simulink library "lib_rigidbody_dynamics_mapletb_mod"  (Simulink 8.5)
settings: Solver=ode45  StartTime=0.0  StopTime=10.0  RelTol=1e-3
undefined symbols (not defined in the file or in its folder): DynPar1, NJ, phi_base_t0, rpy2r, rpyD2omega
undefined symbols (not defined in the file): g_W, KinPar_mdh, phiD_base_t0, r_t0, rD_t0
libraries: transformations_lib x4, rigid_body_kinematics x2
settings Model: Creator=schappler  LastModifiedBy=schappler

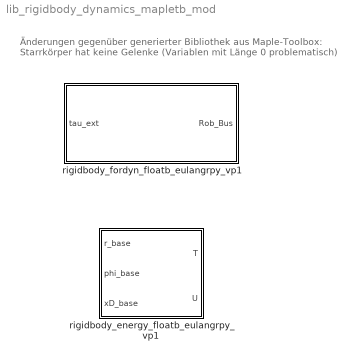
== system lib_rigidbody_dynamics_mapletb_mod ==
  note: Änderungen gegenüber generierter Bibliothek aus Maple-Toolbox:
      | Starrkörper hat keine Gelenke (Variablen mit Länge 0 problematisch)
  rigidbody_energy_floatb_eulangrpy_vp1 : Subsystem  mask{KinPar_mdh=KinPar_mdh, DynPar1=DynPar1, g_world=g_W}
      mask prompts: KinPar_mdh "Kinematik-Parameter"; DynPar1 "Dynamik-Parameter (Parametersatz 1)"; g_world "Gravitationsvektor im Welt-KS (g_world)"
  rigidbody_fordyn_floatb_eulangrpy_vp1 : Subsystem  mask{r_base_t0=r_t0, rD_base_t0=rD_t0, phi_base_t0=phi_base_t0, phiD_base_t0=phiD_base_t0, g_world=g_W, KinPar_mdh=KinPar_mdh, DynPar1=DynPar1}
      mask prompts: r_base_t0 "r_base_t0 (Basisposition im Welt-KS)"; KinPar_mdh "Kinematik-Parameter"; DynPar1 "Dynamik-Parameter (Parametersatz 1)"
      mask Display:
      | port_label('input', 1, '_{(W)} F^{ext}', 'texmode', 'on')
      | port_label('output', 1, 'Rob_Bus')

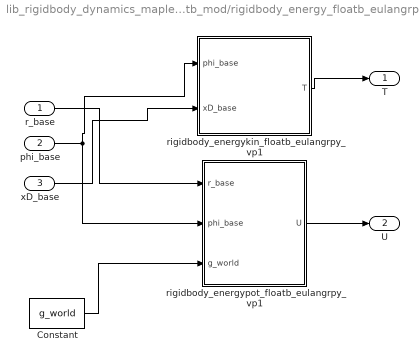
== system lib_rigidbody_dynamics_mapletb_mod/rigidbody_energy_floatb_eulangrpy_vp1 ==
  r_base : Inport
  phi_base : Inport  Port=2
  xD_base : Inport  Port=3
  Constant : Constant  Value=g_world
  rigidbody_energykin_floatb_eulangrpy_vp1 : Subsystem  mask{KinPar_mdh=KinPar_mdh, DynPar1=DynPar1}
      mask prompts: KinPar_mdh "Kinematik-Parameter"; DynPar1 "Dynamik-Parameter (Parametersatz 1)"
      mask init:
      | a_mdh = KinPar_mdh.a;
      | d_mdh = KinPar_mdh.d;
      | b_mdh = KinPar_mdh.b;
      | beta_mdh = KinPar_mdh.beta;
      | alpha_mdh = KinPar_mdh.alpha;
      | q_offset_mdh = KinPar_mdh.q_offset;
      | 
      | m = DynPar1.m;
      | r_S = DynPar1.r_S;
      | I_S = DynPar1.I_S;
  rigidbody_energypot_floatb_eulangrpy_vp1 : Subsystem  mask{KinPar_mdh=KinPar_mdh, DynPar1=DynPar1}
      mask prompts: KinPar_mdh "Kinematik-Parameter"; DynPar1 "Dynamik-Parameter (Parametersatz 1)"
      mask init: same as lib_rigidbody_dynamics_mapletb_mod/rigidbody_energy_floatb_eulangrpy_vp1/rigidbody_energykin_floatb_eulangrpy_vp1
  T : Outport
  U : Outport  Port=2
  wires:
  Constant/1 -> rigidbody_energypot_floatb_eulangrpy_vp1/3(g_world)
  rigidbody_energypot_floatb_eulangrpy_vp1/1(U) -> U/1
  rigidbody_energykin_floatb_eulangrpy_vp1/1(T) -> T/1
  phi_base/1 -> rigidbody_energykin_floatb_eulangrpy_vp1/1(phi_base), rigidbody_energypot_floatb_eulangrpy_vp1/2(phi_base)
  r_base/1 -> rigidbody_energypot_floatb_eulangrpy_vp1/1(r_base)
  xD_base/1 -> rigidbody_energykin_floatb_eulangrpy_vp1/2(xD_base)

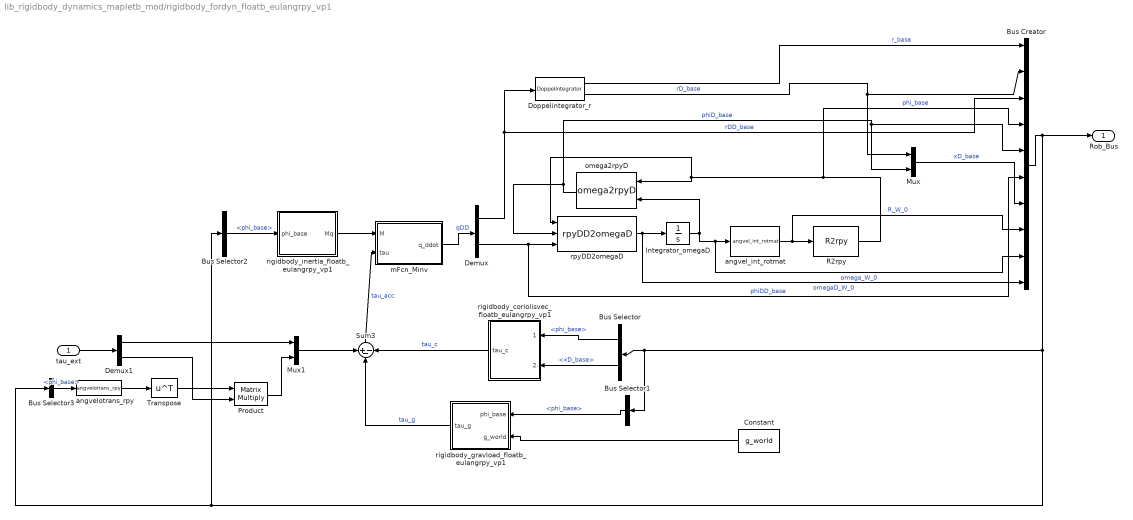
== system lib_rigidbody_dynamics_mapletb_mod/rigidbody_fordyn_floatb_eulangrpy_vp1 ==
  "tau_ext " : Inport  PortDimensions=6+NJ
  Bus Creator : BusCreator  Inputs=10
  Bus Selector : BusSelector  OutputSignals=phi_base,xD_base
  Bus Selector1 : BusSelector  OutputSignals=phi_base
  Bus Selector2 : BusSelector  OutputSignals=phi_base
  Bus Selector3 : BusSelector  OutputSignals=phi_base
  Constant : Constant  Value=g_world
  Demux : Demux  Outputs=[3 3]
  Demux1 : Demux  Outputs=[3 3]
  Doppelintegrator_r : rigid_body_kinematics/Doppelintegrator  r0=r_base_t0  rD0=rD_base_t0  Name_v='x'
  Integrator_omegaD : Integrator  InitialCondition=rpyD2omega(phi_base_t0', phiD_base_t0')'
  Mux : Mux  Inputs=2
  Mux1 : Mux  Inputs=2
  Product : Product  Multiplication=Matrix(*)
  R2rpy : transformations_lib/R2rpy
  Sum3 : Sum  Inputs=+--
  Transpose : Math  Operator=transpose  SaturateOnIntegerOverflow=on
  angvel_int_rotmat : rigid_body_kinematics/angvel_int_rotmat  R_0E_t0=rpy2r(phi_base_t0(1), phi_base_t0(2), phi_base_t0(3) )
  angvelotrans_rpy : transformations_lib/angvelotrans_rpy
  mFcn_Minv : MATLAB Function  TreatAsAtomicUnit=on
  omega2rpyD : transformations_lib/omega2rpyD
  rigidbody_coriolisvec_floatb_eulangrpy_vp1 : Subsystem  mask{KinPar_mdh=KinPar_mdh, DynPar1=DynPar1}
      mask prompts: KinPar_mdh "Kinematik-Parameter"; DynPar1 "Dynamik-Parameter (Parametersatz 1)"
      mask init: same as lib_rigidbody_dynamics_mapletb_mod/rigidbody_energy_floatb_eulangrpy_vp1/rigidbody_energykin_floatb_eulangrpy_vp1
  rigidbody_gravload_floatb_eulangrpy_vp1 : Subsystem  mask{KinPar_mdh=KinPar_mdh, DynPar1=DynPar1}
      mask prompts: KinPar_mdh "Kinematik-Parameter"; DynPar1 "Dynamik-Parameter (Parametersatz 1)"
      mask init: same as lib_rigidbody_dynamics_mapletb_mod/rigidbody_energy_floatb_eulangrpy_vp1/rigidbody_energykin_floatb_eulangrpy_vp1
  rigidbody_inertia_floatb_eulangrpy_vp1 : Subsystem  mask{KinPar_mdh=KinPar_mdh, DynPar1=DynPar1}
      mask prompts: KinPar_mdh "Kinematik-Parameter"; DynPar1 "Dynamik-Parameter (Parametersatz 1)"
      mask init: same as lib_rigidbody_dynamics_mapletb_mod/rigidbody_energy_floatb_eulangrpy_vp1/rigidbody_energykin_floatb_eulangrpy_vp1
  rpyDD2omegaD : transformations_lib/rpyDD2omegaD
  Rob_Bus : Outport
  wires:
  Bus Selector2/1 -> rigidbody_inertia_floatb_eulangrpy_vp1/1(phi_base)  "<phi_base>"
  Bus Selector1/1 -> rigidbody_gravload_floatb_eulangrpy_vp1/1(phi_base)  "<phi_base>"
  Bus Selector/1 -> rigidbody_coriolisvec_floatb_eulangrpy_vp1/1(phi_base)  "<phi_base>"
  Bus Selector/2 -> rigidbody_coriolisvec_floatb_eulangrpy_vp1/2(xD_base)  "<xD_base>"
  Bus Creator/1 -> Rob_Bus/1, Bus Selector/1, Bus Selector1/1, Bus Selector3/1, Bus Selector2/1
  Mux/1 -> Bus Creator/7  "xD_base"
  Doppelintegrator_r/2 -> Bus Creator/2, Mux/1  "rD_base"
  Doppelintegrator_r/1 -> Bus Creator/1  "r_base"
  omega2rpyD/1 -> Bus Creator/5, Mux/2, rpyDD2omegaD/2  "phiD_base"
  R2rpy/1 -> omega2rpyD/1, rpyDD2omegaD/1, Bus Creator/4  "phi_base"
  angvel_int_rotmat/1 -> Bus Creator/8, R2rpy/1  "R_W_0"
  Demux/2 -> Bus Creator/6, rpyDD2omegaD/3  "phiDD_base"
  Integrator_omegaD/1 -> Bus Creator/9, angvel_int_rotmat/1, omega2rpyD/2  "omega_W_0"
  rpyDD2omegaD/1 -> Integrator_omegaD/1, Bus Creator/10  "omegaD_W_0"
  Demux/1 -> Doppelintegrator_r/1, Bus Creator/3  "rDD_base"
  rigidbody_gravload_floatb_eulangrpy_vp1/1(tau_g) -> Sum3/2  "tau_g"
  mFcn_Minv/1(q_ddot) -> Demux/1  "qDD"
  rigidbody_coriolisvec_floatb_eulangrpy_vp1/1(tau_c) -> Sum3/3  "tau_c"
  "tau_ext "/1 -> Demux1/1
  Sum3/1 -> mFcn_Minv/2(tau)  "tau_acc"
  rigidbody_inertia_floatb_eulangrpy_vp1/1(Mq) -> mFcn_Minv/1(M)
  Constant/1 -> rigidbody_gravload_floatb_eulangrpy_vp1/2(g_world)
  Demux1/2 -> Product/2
  Demux1/1 -> Mux1/1
  Bus Selector3/1 -> angvelotrans_rpy/1  "<phi_base>"
  angvelotrans_rpy/1 -> Transpose/1
  Product/1 -> Mux1/2
  Mux1/1 -> Sum3/1
  Transpose/1 -> Product/1

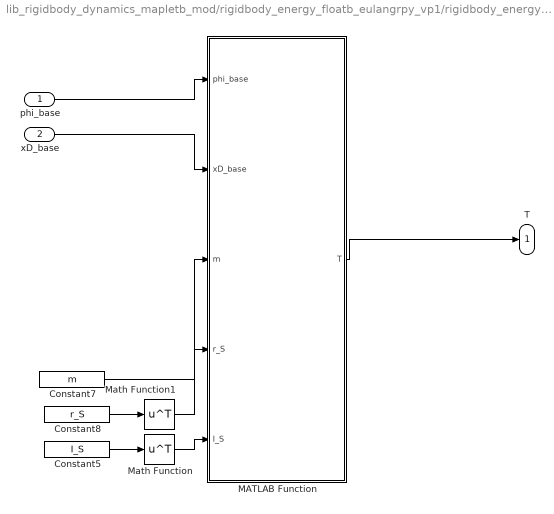
== system lib_rigidbody_dynamics_mapletb_mod/rigidbody_energy_floatb_eulangrpy_vp1/rigidbody_energykin_floatb_eulangrpy_vp1 ==
  phi_base : Inport
  xD_base : Inport  Port=2
  Constant5 : Constant  Value=I_S
  Constant7 : Constant  Value=m
  Constant8 : Constant  Value=r_S
  MATLAB Function : MATLAB Function  TreatAsAtomicUnit=on
  Math Function : Math  Operator=transpose  SaturateOnIntegerOverflow=on
  Math Function1 : Math  Operator=transpose  SaturateOnIntegerOverflow=on
  T : Outport
  wires:
  xD_base/1 -> MATLAB Function/2(xD_base)
  phi_base/1 -> MATLAB Function/1(phi_base)
  Constant5/1 -> Math Function/1
  Constant8/1 -> Math Function1/1
  Constant7/1 -> MATLAB Function/3(m)
  MATLAB Function/1(T) -> T/1
  Math Function/1 -> MATLAB Function/5(I_S)
  Math Function1/1 -> MATLAB Function/4(r_S)

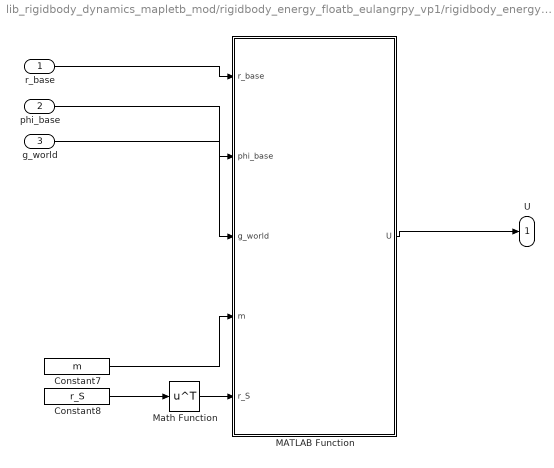
== system lib_rigidbody_dynamics_mapletb_mod/rigidbody_energy_floatb_eulangrpy_vp1/rigidbody_energypot_floatb_eulangrpy_vp1 ==
  r_base : Inport
  phi_base : Inport  Port=2
  g_world : Inport  Port=3
  Constant7 : Constant  Value=m
  Constant8 : Constant  Value=r_S
  MATLAB Function : MATLAB Function  TreatAsAtomicUnit=on
  Math Function : Math  Operator=transpose  SaturateOnIntegerOverflow=on
  U : Outport
  wires:
  phi_base/1 -> MATLAB Function/2(phi_base)
  r_base/1 -> MATLAB Function/1(r_base)
  Constant8/1 -> Math Function/1
  Constant7/1 -> MATLAB Function/4(m)
  g_world/1 -> MATLAB Function/3(g_world)
  MATLAB Function/1(U) -> U/1
  Math Function/1 -> MATLAB Function/5(r_S)

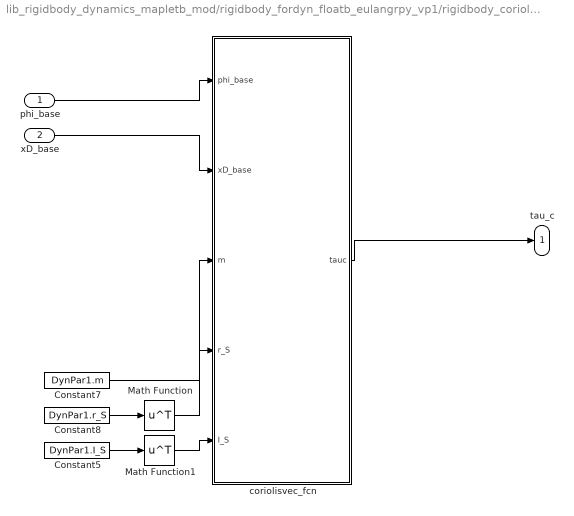
== system lib_rigidbody_dynamics_mapletb_mod/rigidbody_fordyn_floatb_eulangrpy_vp1/rigidbody_coriolisvec_floatb_eulangrpy_vp1 ==
  phi_base : Inport
  xD_base : Inport  Port=2
  Constant5 : Constant  Value=DynPar1.I_S
  Constant7 : Constant  Value=DynPar1.m
  Constant8 : Constant  Value=DynPar1.r_S
  Math Function : Math  Operator=transpose  SaturateOnIntegerOverflow=on
  Math Function1 : Math  Operator=transpose  SaturateOnIntegerOverflow=on
  coriolisvec_fcn : MATLAB Function  TreatAsAtomicUnit=on
  tau_c : Outport
  wires:
  xD_base/1 -> coriolisvec_fcn/2(xD_base)
  phi_base/1 -> coriolisvec_fcn/1(phi_base)
  Constant5/1 -> Math Function1/1
  Constant8/1 -> Math Function/1
  Constant7/1 -> coriolisvec_fcn/3(m)
  coriolisvec_fcn/1(tauc) -> tau_c/1
  Math Function/1 -> coriolisvec_fcn/4(r_S)
  Math Function1/1 -> coriolisvec_fcn/5(I_S)

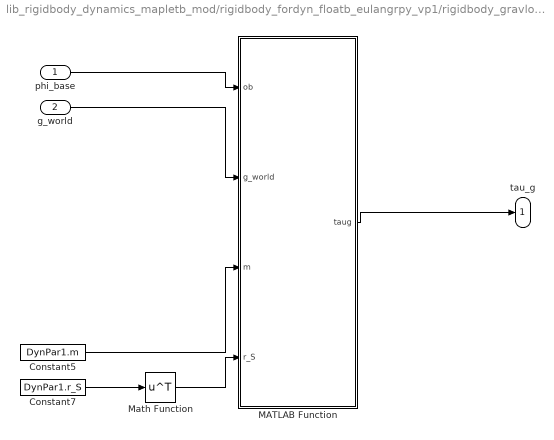
== system lib_rigidbody_dynamics_mapletb_mod/rigidbody_fordyn_floatb_eulangrpy_vp1/rigidbody_gravload_floatb_eulangrpy_vp1 ==
  phi_base : Inport
  g_world : Inport  Port=2
  Constant5 : Constant  Value=DynPar1.m
  Constant7 : Constant  Value=DynPar1.r_S
  MATLAB Function : MATLAB Function  TreatAsAtomicUnit=on
  Math Function : Math  Operator=transpose  SaturateOnIntegerOverflow=on
  tau_g : Outport
  wires:
  phi_base/1 -> MATLAB Function/1(ob)
  Constant7/1 -> Math Function/1
  Constant5/1 -> MATLAB Function/3(m)
  g_world/1 -> MATLAB Function/2(g_world)
  MATLAB Function/1(taug) -> tau_g/1
  Math Function/1 -> MATLAB Function/4(r_S)

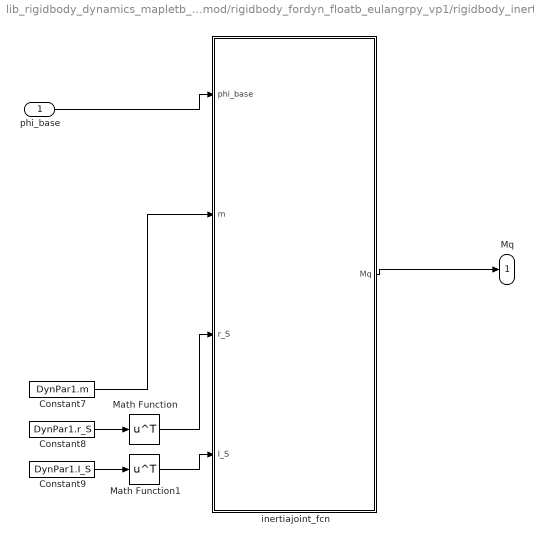
== system lib_rigidbody_dynamics_mapletb_mod/rigidbody_fordyn_floatb_eulangrpy_vp1/rigidbody_inertia_floatb_eulangrpy_vp1 ==
  phi_base : Inport
  Constant7 : Constant  Value=DynPar1.m
  Constant8 : Constant  Value=DynPar1.r_S
  Constant9 : Constant  Value=DynPar1.I_S
  Math Function : Math  Operator=transpose  SaturateOnIntegerOverflow=on
  Math Function1 : Math  Operator=transpose  SaturateOnIntegerOverflow=on
  inertiajoint_fcn : MATLAB Function  TreatAsAtomicUnit=on
  Mq : Outport
  wires:
  phi_base/1 -> inertiajoint_fcn/1(phi_base)
  Constant9/1 -> Math Function1/1
  Constant8/1 -> Math Function/1
  inertiajoint_fcn/1(Mq) -> Mq/1
  Constant7/1 -> inertiajoint_fcn/2(m)
  Math Function/1 -> inertiajoint_fcn/3(r_S)
  Math Function1/1 -> inertiajoint_fcn/4(I_S)

== matlab function rigidbody_fordyn_floatb_eulangrpy_vp1/rigidbody_gravload_floatb_eulangrpy_vp1/MATLAB Function ==
  data: taug output double; ob input double; g_world input double; m input double; r_S input double
function taug = gravload(ob, g_world, ...
  m, r_S)
%#codegen
q = zeros(0,1);
alpha_mdh = zeros(0,1);
a_mdh = zeros(0,1);
d_mdh = zeros(0,1);
q_offset_mdh = zeros(0,1);
b_mdh = zeros(0,1);
beta_mdh = zeros(0,1);
taug_base = rigidbody_gravload_base_floatb_eulangrpy_slag_vp1(q, ob, g_world, ...
  alpha_mdh, a_mdh, d_mdh, q_offset_mdh, b_mdh, beta_mdh, m, r_S);
taug = [taug_base];

== matlab function rigidbody_fordyn_floatb_eulangrpy_vp1/rigidbody_coriolisvec_floatb_eulangrpy_vp1/coriolisvec_fcn ==
  data: tauc output double; phi_base input double; xD_base input double; m input double; r_S input double; I_S input double
function tauc = coriolis(phi_base, xD_base, ...
   m, r_S, I_S)
%#codegen
q = zeros(0,1);
qD = zeros(0,1);
alpha_mdh = zeros(0,1);
a_mdh = zeros(0,1);
d_mdh = zeros(0,1);
q_offset_mdh = zeros(0,1);
b_mdh = zeros(0,1);
beta_mdh = zeros(0,1);
tauc = rigidbody_coriolisvec_floatb_eulangrpy_slag_vp1(q, qD, phi_base, xD_base, ...
  alpha_mdh, a_mdh, d_mdh, q_offset_mdh, b_mdh, beta_mdh, m, r_S, I_S);

== matlab function rigidbody_fordyn_floatb_eulangrpy_vp1/rigidbody_inertia_floatb_eulangrpy_vp1/inertiajoint_fcn ==
  data: phi_base input double; Mq output double; m input double; r_S input double; I_S input double
function Mq = inertia(phi_base, ...
  m, r_S, I_S)
%#codegen
q = zeros(0,1);

alpha_mdh = zeros(0,1);
a_mdh = zeros(0,1);
d_mdh = zeros(0,1);
q_offset_mdh = zeros(0,1);
b_mdh = zeros(0,1);
beta_mdh = zeros(0,1);
Mq = rigidbody_inertia_floatb_eulangrpy_slag_vp1(q, phi_base, ...
  alpha_mdh, a_mdh, d_mdh, q_offset_mdh, b_mdh, beta_mdh, m, r_S, I_S);

== matlab function rigidbody_energy_floatb_eulangrpy_vp1/rigidbody_energypot_floatb_eulangrpy_vp1/MATLAB Function ==
  data: U output double; r_base input double; phi_base input double; g_world input double; m input double; r_S input double
function U = energypot(r_base, phi_base, g_world, ...
  m, r_S)

q = zeros(0,1);
alpha_mdh = zeros(0,1);
a_mdh = zeros(0,1);
d_mdh = zeros(0,1);
q_offset_mdh = zeros(0,1);
b_mdh = zeros(0,1);
beta_mdh = zeros(0,1);

%#codegen
U = rigidbody_energypot_floatb_eulangrpy_slag_vp1(q, r_base, phi_base, g_world, ...
  alpha_mdh, a_mdh, d_mdh, q_offset_mdh, b_mdh, beta_mdh, m, r_S);

== matlab function rigidbody_energy_floatb_eulangrpy_vp1/rigidbody_energykin_floatb_eulangrpy_vp1/MATLAB Function ==
  data: T output double; phi_base input double; xD_base input double; m input double; r_S input double; I_S input double
function T = energykin(phi_base, xD_base,  ...
  m, r_S, I_S)

q = zeros(0,1);
qD = zeros(0,1);
alpha_mdh = zeros(0,1);
a_mdh = zeros(0,1);
d_mdh = zeros(0,1);
q_offset_mdh = zeros(0,1);
b_mdh = zeros(0,1);
beta_mdh = zeros(0,1);

%#codegen
T = rigidbody_energykin_floatb_eulangrpy_slag_vp1(q, qD, phi_base, xD_base, ...
  alpha_mdh, a_mdh, d_mdh, q_offset_mdh, b_mdh, beta_mdh, m, r_S, I_S);

== matlab function rigidbody_fordyn_floatb_eulangrpy_vp1/mFcn_Minv ==
  data: M input double; q_ddot output double; tau input double
function q_ddot = fcn(M,tau)
%#codegen
q_ddot=M\tau;
